simulink subsystem "GetTransformEE"  (R2022a)
settings: Solver=VariableStepAuto  StartTime=0.0  StopTime=10.0  RelTol=1e-3
model mask{spaceRobot=0}
settings Model: Creator=charl  LastModifiedBy=charl

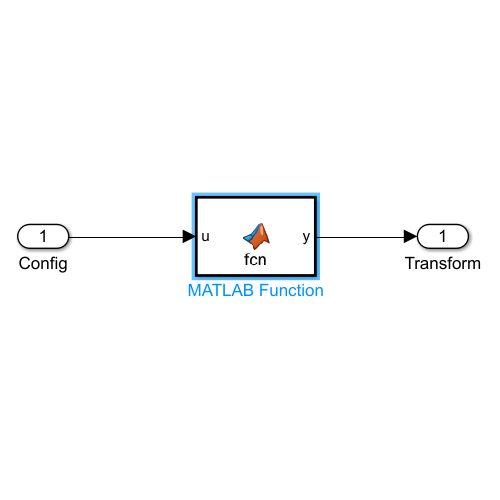
[thumbnail: Simulink's stored preview of the top-level diagram]
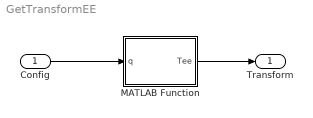
== system GetTransformEE ==
  Config : Inport
  MATLAB Function : MATLAB Function  TreatAsAtomicUnit=on
  Transform : Outport  VectorParamsAs1DForOutWhenUnconnected=off
  wires:
  Config/1 -> MATLAB Function/1(q)
  MATLAB Function/1(Tee) -> Transform/1

== matlab function GetTransformEE/MATLAB Function ==
  data: q input; Tee output
function Tee = fcn(q)
[~, ~, ~, Tee] = RFunc_SR2(q);
